simulink subsystem "Controller"  (R2023b)
settings: Solver=VariableStepAuto  StartTime=0.0  StopTime=10.0  RelTol=1e-3
undefined symbols (not defined in the file or in its folder): m1, m2, m3, V1, V2, V3
libraries: dspinverses x2, aerolibutil x2, sharedtransform x2, matrix_library x1
settings Model: Creator=andrea  LastModifiedBy=andrea

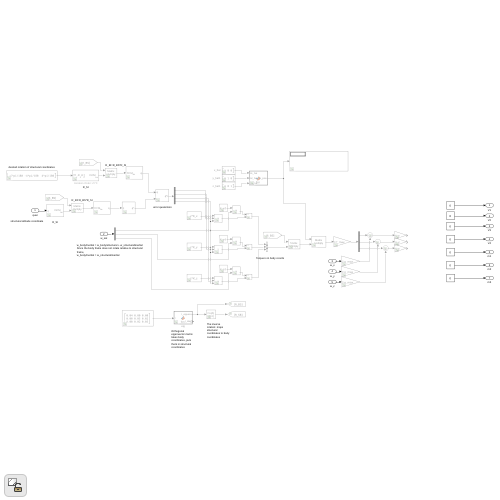
[thumbnail: Simulink's stored preview of the top-level diagram]
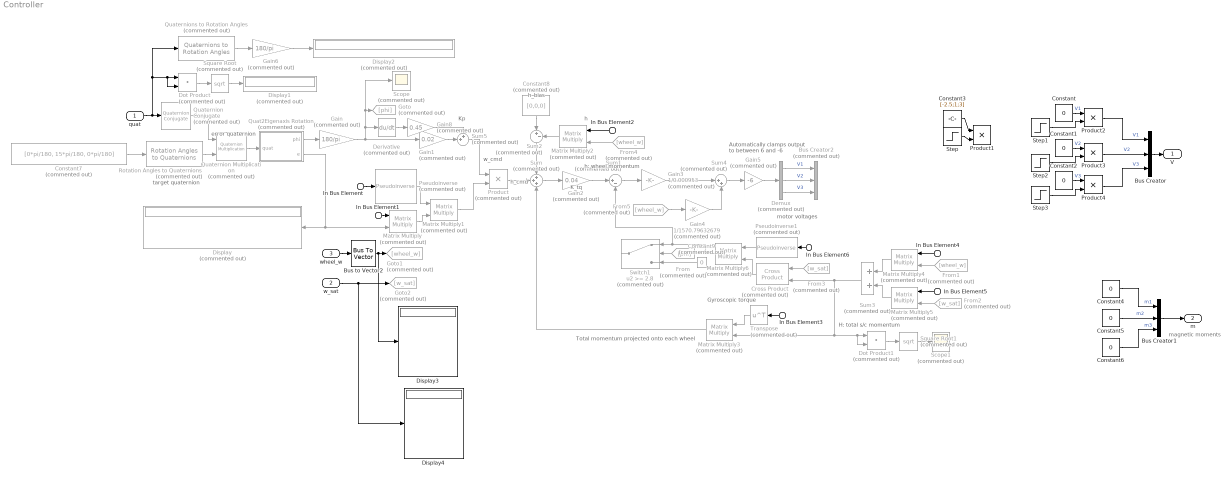
== system Controller ==
  note: Automatically clamps output to between 6 and -6
  note: Total momentum projected onto each wheel
  note: Gyroscopic torque
  note: H: total s/c momentum
  note: h: wheel momentum
  note: h_bias
  note: h
  note: h_cmd
  note: w_cmd
  note: Kp
  note: magnetic moments
  note: motor voltages
  note: target quaternion
  note: error quaternion
  note: K_tq
  quat : Inport  PortDimensions=4
  w_sat : Inport  Port=2  PortDimensions=3
  wheel_w : Inport  Port=3
  In Bus Element : Inport  Port=4  PortName=Params  Element=A
  In Bus Element3 : Inport  Port=4  PortName=Params  Element=A
  In Bus Element6 : Inport  Port=4  PortName=Params  Element=A
  In Bus Element1 : Inport  Port=4  PortName=Params  Element=I_sat
  In Bus Element5 : Inport  Port=4  PortName=Params  Element=I_sat
  In Bus Element2 : Inport  Port=4  PortName=Params  Element=I_wheels
  In Bus Element4 : Inport  Port=4  PortName=Params  Element=I_wheels
  Bus Creator : BusCreator  Inputs=3
  Bus Creator1 : BusCreator  Inputs=m1,m2,m3
  Bus Creator2 : BusCreator  Commented=on  Inputs=V1,V2,V3
  Bus to Vector2 : BusToVector
  Constant{,1..2,4..6} (6 alike) : Constant  Value=0
  Constant3 : Constant  Value=[-2.5;1;3]
  Constant7 : Constant  Commented=on  Value=[0*pi/180, 15*pi/180, 0*pi/180]  VectorParams1D=off
  Constant8 : Constant  Commented=on  Value=[0,0,0]
  Constant9 : Constant  Commented=on  Value=0
  Cross Product : matrix_library/Cross Product  Commented=on
  Demux : Demux  Commented=on  Outputs=3
  Derivative : Derivative  Commented=on
  Display : Display  Commented=on
  Display1 : Display  Commented=on
  Display2 : Display  Commented=on
  Display3 : Display
  Display4 : Display
  Dot Product : DotProduct  Commented=on  OutDataTypeStr=Inherit: Inherit via internal rule
  Dot Product1 : DotProduct  Commented=on  OutDataTypeStr=Inherit: Inherit via internal rule
  From : From  Commented=on  GotoTag=phi
  From1 : From  Commented=on  GotoTag=wheel_w
  From2 : From  Commented=on  GotoTag=w_sat
  From3 : From  Commented=on  GotoTag=w_sat
  From4 : From  Commented=on  GotoTag=wheel_w
  From5 : From  Commented=on  GotoTag=wheel_w
  Gain : Gain  Commented=on  Gain=180/pi
  Gain1 : Gain  Commented=on  Gain=0.02
  Gain2 : Gain  Commented=on  Gain=0.04
  Gain3 : Gain  Commented=on  Gain=1/0.000953
  Gain4 : Gain  Commented=on  Gain=1/1570.79632679
  Gain5 : Gain  Commented=on  Gain=-6  OutMin=-6  OutMax=6
  Gain6 : Gain  Commented=on  Gain=180/pi
  Gain8 : Gain  Commented=on  Gain=0.45
  Goto : Goto  Commented=on  GotoTag=phi
  Goto1 : Goto  Commented=on  GotoTag=wheel_w
  Goto2 : Goto  Commented=on  GotoTag=w_sat
  Matrix Multiply{,1..6} (7 alike) : Product  Commented=on  Multiplication=Matrix(*)
  Product : Product  Commented=on
  Product{1..4} (4 alike) : Product
  Pseudoinverse : dspinverses/Pseudoinverse  Commented=on  wanterr=off  SimulateUsing=Interpreted execution
  Pseudoinverse1 : dspinverses/Pseudoinverse  Commented=on  wanterr=off  SimulateUsing=Interpreted execution
  Quat2Eigenaxis Rotation : MATLAB Function  Commented=on  TreatAsAtomicUnit=on
  Quaternion Conjugate : aerolibutil/Quaternion Conjugate  Commented=on
  Quaternion Multiplication : aerolibutil/Quaternion Multiplication  Commented=on
  Quaternions to Rotation Angles : sharedtransform/Quaternions to Rotation Angles  Commented=on  rotationOrder=ZYX  aMode=aMode
  Rotation Angles to Quaternions : sharedtransform/Rotation Angles to Quaternions  Commented=on  rotationOrder=ZYX  aMode=aMode
  Scope : Scope  Commented=on
  Scope1 : Scope  Commented=on
  Square Root : Sqrt  Commented=on
  Square Root1 : Sqrt  Commented=on
  Step : Step  Before=1  After=-1  SampleTime=0
  Step1 : Step  Time=2  Before=1  After=-1  SampleTime=0
  Step2 : Step  Time=2  Before=1  After=-1  SampleTime=0
  Step3 : Step  Time=2  Before=1  After=-1  SampleTime=0
  Sum : Sum  Commented=on  Inputs=+++
  Sum1 : Sum  Commented=on  Inputs=|+-
  Sum2 : Sum  Commented=on  Inputs=|+-
  Sum3 : Sum  Commented=on
  Sum4 : Sum  Commented=on  Inputs=|++
  Sum5 : Sum  Commented=on  Inputs=++|
  Switch1 : Switch  Commented=on  Threshold=2.8  SaturateOnIntegerOverflow=off  InputSameDT=off
  Transpose : Math  Commented=on  Operator=transpose
  V : Outport
  m : Outport  Port=2
  wires:
  quat/1 -> Quaternion Conjugate/1, Quaternions to Rotation Angles/1, Dot Product/1, Dot Product/2
  Quaternion Multiplication/1 -> Quat2Eigenaxis Rotation/1(quat)
  Constant7/1 -> Rotation Angles to Quaternions/1
  Rotation Angles to Quaternions/1 -> Quaternion Multiplication/2
  Quaternion Conjugate/1 -> Quaternion Multiplication/1
  Quat2Eigenaxis Rotation/1(phi) -> Gain/1
  Gain/1 -> Derivative/1, Goto/1, Scope/1, Gain1/1
  Constant5/1 -> Bus Creator1/2  "m2"
  Bus Creator1/1 -> m/1
  Constant6/1 -> Bus Creator1/3  "m3"
  Constant4/1 -> Bus Creator1/1  "m1"
  In Bus Element/1 -> Pseudoinverse/1
  Pseudoinverse/1 -> Matrix Multiply1/1
  Matrix Multiply/1 -> Matrix Multiply1/2
  Matrix Multiply1/1 -> Product/2
  Product/1 -> Sum/2
  Gain2/1 -> Sum1/1
  Sum/1 -> Gain2/1
  In Bus Element2/1 -> Matrix Multiply2/1
  From4/1 -> Matrix Multiply2/2
  Sum2/1 -> Sum/1
  Matrix Multiply2/1 -> Sum2/2
  Constant8/1 -> Sum2/1
  In Bus Element3/1 -> Transpose/1
  Transpose/1 -> Matrix Multiply3/1
  In Bus Element4/1 -> Matrix Multiply4/1
  From1/1 -> Matrix Multiply4/2
  Matrix Multiply4/1 -> Sum3/1
  Matrix Multiply5/1 -> Sum3/2
  In Bus Element5/1 -> Matrix Multiply5/1
  wheel_w/1 -> Bus to Vector2/1
  Bus to Vector2/1 -> Goto1/1, Display3/1
  w_sat/1 -> Goto2/1, Display4/1
  From2/1 -> Matrix Multiply5/2
  From3/1 -> Cross Product/1
  Sum3/1 -> Cross Product/2, Matrix Multiply3/2, Dot Product1/1, Dot Product1/2
  From/1 -> Switch1/2
  Constant9/1 -> Switch1/3
  Sum1/1 -> Gain3/1
  From5/1 -> Gain4/1
  Gain3/1 -> Sum4/1
  Gain4/1 -> Sum4/2
  Sum4/1 -> Gain5/1
  Gain5/1 -> Demux/1
  Demux/1 -> Bus Creator2/1  "V1"
  Demux/2 -> Bus Creator2/2  "V2"
  Demux/3 -> Bus Creator2/3  "V3"
  In Bus Element1/1 -> Matrix Multiply/1
  Quat2Eigenaxis Rotation/2(e) -> Display/1, Matrix Multiply/2
  In Bus Element6/1 -> Pseudoinverse1/1
  Cross Product/1 -> Matrix Multiply6/2
  Pseudoinverse1/1 -> Matrix Multiply6/1
  Matrix Multiply6/1 -> Switch1/1, Sum1/2
  Dot Product/1 -> Square Root/1
  Square Root/1 -> Display1/1
  Gain6/1 -> Display2/1
  Quaternions to Rotation Angles/1 -> Gain6/1
  Gain1/1 -> Sum5/2
  Sum5/1 -> Product/1
  Derivative/1 -> Gain8/1
  Gain8/1 -> Sum5/1
  Matrix Multiply3/1 -> Sum/3
  Dot Product1/1 -> Square Root1/1
  Square Root1/1 -> Scope1/1
  Bus Creator/1 -> V/1
  Step/1 -> Product1/2
  Constant3/1 -> Product1/1
  Step1/1 -> Product2/2
  Constant/1 -> Product2/1  "V1"
  Step2/1 -> Product3/2
  Constant1/1 -> Product3/1  "V2"
  Step3/1 -> Product4/2
  Constant2/1 -> Product4/1  "V3"
  Product4/1 -> Bus Creator/3  "V3"
  Product3/1 -> Bus Creator/2  "V2"
  Product2/1 -> Bus Creator/1  "V1"

== matlab function Controller/Quat2Eigenaxis Rotation ==
  data: quat input; phi output; e output
function [phi, e] = fcn(quat)

e = [0;0;0];
phi = 0;

coder.extrinsic("quat2axang");
axang = quat2axang(reshape(quat,[1,4]));
%e = [axang(1,1), axang(1,2), axang(1,3)];
e = reshape([axang(1,1), axang(1,2), axang(1,3)],[3,1]);
phi = axang(1,4);


%e = reshape(e,[3,1]);

%e = [axang(0,1); axang(0,2); axang(0,3)];
%phi = axang(0,4);
